simulink model "multi_rotor_sim"  (R2023b)
settings: Solver=ode4  StartTime=0.0  StopTime=inf  FixedStep=ST  RelTol=1e-3
values from neighbouring files (symbols this model uses):
  a0 = 0    [parameters.m]
  ASLOPE = 5.9    [parameters.m]
  Ax = 0.023    [parameters.m]
  Ay = 0.023    [parameters.m]
  Az = 0.106    [parameters.m]
  BLADES = 2    [parameters.m]
  BLCG = 0    [parameters.m]
  BLCP = 0    [parameters.m]
  BLH1 = b*sind(30)    [parameters.m]
  BLH2 = b    (= 0.275)    [parameters.m]
  BLH3 = b*sind(30)    [parameters.m]
  BLH4 = -b*sind(30)    [parameters.m]
  BLH5 = -b    (= -0.275)    [parameters.m]
  BLH6 = -b*sind(30)    [parameters.m]
  chi1 = 1    [parameters.m]
  chi2 = -1    [parameters.m]
  chi3 = 1    [parameters.m]
  chi4 = -1    [parameters.m]
  chi5 = 1    [parameters.m]
  chi6 = -1    [parameters.m]
  CHORD = 17.55e-3    (= 0.01755)    [parameters.m]
  CHORD75 = 21e-3    (= 0.021)    [parameters.m]
  dyn_viscosity = 17.89e-6    (= 1.789e-05)    [parameters.m]
  g0 = 9.80665    [parameters.m]
  href = 0    [parameters.m]
  k_ind = 1.35    [parameters.m]
  k_Omega = 14.92    [parameters.m]
  latref = 44.200626    [parameters.m]
  lonref = 12.063822    [parameters.m]
  m = 2.15    [parameters.m]
  MC_ATT_PITCH = 45*pi/180    (= 0.785398163397)    [parameters.m]
  MC_ATT_ROLL = 45*pi/180    (= 0.785398163397)    [parameters.m]
  MC_PITCH_P = 2    [parameters.m]
  MC_PITCHRATE_D = 0    [parameters.m]
  MC_PITCHRATE_I = 0.05    [parameters.m]
  MC_PITCHRATE_P = 0.09*3    (= 0.27)    [parameters.m]
  MC_RATE_PITCH = 500*pi/180    (= 8.72664625997)    [parameters.m]
  MC_RATE_ROLL = 500*pi/180    (= 8.72664625997)    [parameters.m]
  MC_RATE_YAW = 300*pi/180    (= 5.23598775598)    [parameters.m]
  MC_ROLL_P = 2    [parameters.m]
  MC_ROLLRATE_D = 0    [parameters.m]
  MC_ROLLRATE_I = 0.05    [parameters.m]
  MC_ROLLRATE_P = 0.09*3    (= 0.27)    [parameters.m]
  MC_VEL_FWD = 15    [parameters.m]
  MC_VEL_FWD_OPT = 0.5    [parameters.m]
  MC_VEL_LAT = 15    [parameters.m]
  MC_VEL_LAT_OPT = 0.5    [parameters.m]
  MC_VEL_VERT = 15    [parameters.m]
  MC_YAW_P = 0.55    [parameters.m]
  MC_YAWRATE_D = 0.05    [parameters.m]
  MC_YAWRATE_I = 0.02    [parameters.m]
  MC_YAWRATE_P = 0.15*3    (= 0.45)    [parameters.m]
  MPC_XY_VEL_D_ACC = 0.6    [parameters.m]
  MPC_XY_VEL_I_ACC = 0.8    [parameters.m]
  MPC_XY_VEL_P_ACC = 1.7    [parameters.m]
  MPC_Z_VEL_D_ACC = 0    [parameters.m]
  MPC_Z_VEL_I_ACC = 2    [parameters.m]
  MPC_Z_VEL_P_ACC = 4    [parameters.m]
  n = 0.6359    [parameters.m]
  p00 = 7.145e-2    (= 0.07145)    [parameters.m]
  p01 = 0.4377    [parameters.m]
  p02 = -10.13    [parameters.m]
  p10 = 1.259e-3    (= 0.001259)    [parameters.m]
  p11 = 1.284e-3    (= 0.001284)    [parameters.m]
  p20 = -7.513e-7    (= -7.513e-07)    [parameters.m]
  PWM_hover = (PWM_idle+PWM_max)/2    (= 1550)    [parameters.m]
  PWM_idle = 1100    [parameters.m]
  PWM_max = 2000    [parameters.m]
  ROTOR = 4*0.0254    (= 0.1016)    [parameters.m]
  ST = 0.01    [parameters.m]
  STACG = 0    [parameters.m]
  STACP = 0    [parameters.m]
  STAH1 = -b*cosd(30)    [parameters.m]
  STAH2 = 0    [parameters.m]
  STAH3 = b*cosd(30)    [parameters.m]
  STAH4 = b*cosd(30)    [parameters.m]
  STAH5 = 0    [parameters.m]
  STAH6 = -b*cosd(30)    [parameters.m]
  TERMINAL_SPEED = 0.5    [parameters.m]
  Theta0 = 45*pi/180    (= 0.785398163397)    [parameters.m]
  THETT = -38.0973*pi/180    (= -0.66492332112)    [parameters.m]
  wind_rate = [ 0 0 0 ]'    [parameters.m]
  wind_velocity_e = [ 0 0 0 ]'    [parameters.m]
  WLCG = -0.02    [parameters.m]
  WLCP = -0.08    [parameters.m]
  WLH1 = 32e-3    (= 0.032)    [parameters.m]
  WLH2 = 32e-3    (= 0.032)    [parameters.m]
  WLH3 = 32e-3    (= 0.032)    [parameters.m]
  WLH4 = 32e-3    (= 0.032)    [parameters.m]
  WLH5 = 32e-3    (= 0.032)    [parameters.m]
  WLH6 = 32e-3    (= 0.032)    [parameters.m]
undefined symbols (not defined in the file or in its folder): Earth, WGS84, X, Y, Z
libraries: sm_lib x258, slpidlib x36, nesl_utility x15, sharedtransform x13, aerolibutil x4, aerolibanimutils x3, sharedutil x2, sim3dlib x1, uavsim3dlib x1, shared6dof x1, aerolibtransform2 x1, aerolibatmos2 x1
(part 2 of 11)

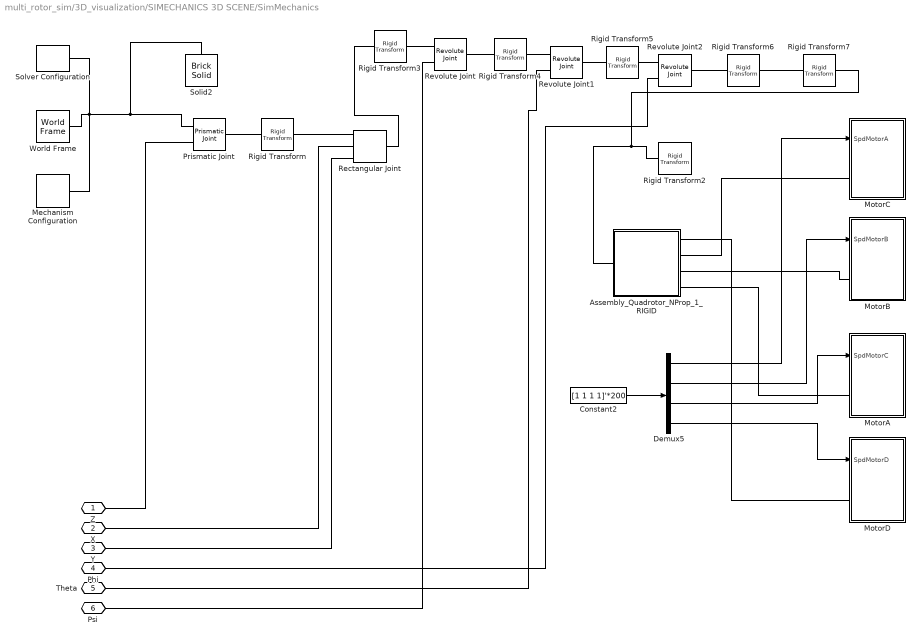
== system multi_rotor_sim/3D_visualization/SIMECHANICS 3D SCENE/SimMechanics ==
  Assembly_Quadrotor_NProp_1_RIGID : Subsystem
  Constant2 : Constant  Value=[1 1 1 1]'*200
  Demux5 : Demux
  Mechanism Configuration : sm_lib/Utilities/Mechanism Configuration  UniformGravity=Constant  GravityVector=[0 0 9.80665]  GravityVectorUnits=m/s^2  LinearizationDelta=0.001  JointModeTransitionNonlinearIterations=2
  MotorA : Subsystem
  MotorB : Subsystem
  MotorC : Subsystem
  MotorD : Subsystem
  Prismatic Joint : sm_lib/Joints/Prismatic Joint  JointMode=Normal  SenseConstraintForce=off  SenseConstraintForceX=off  SenseConstraintForceY=off  SenseConstraintForceZ=off  SenseConstraintTorque=off  SenseConstraintTorqueX=off  SenseConstraintTorqueY=off  SenseConstraintTorqueZ=off  SenseTotalForce=off  SenseTotalForceX=off  SenseTotalForceY=off  SenseTotalForceZ=off  SenseTotalTorque=off  SenseTotalTorqueX=off  SenseTotalTorqueY=off  SenseTotalTorqueZ=off  CompositeWrenchDir=FollowerOnBase  CompositeWrenchFrame=BaseFrame  EquilibriumPosition=0  EquilibriumPositionUnits=m  SpringStiffness=0  SpringStiffnessUnits=N/m  DampingCoefficient=0  DampingCoefficientUnits=N/(m/s)  TorqueActuationMode=ComputedTorque  MotionActuationMode=InputMotion  SensePosition=off  SenseVelocity=off  SenseAcceleration=off  SenseTorqueForce=off  SenseLowerLimitTorqueForce=off  SenseUpperLimitTorqueForce=off  LowerLimitSpecify=off  LowerLimitBound=-1  LowerLimitBoundUnits=m  LowerLimitStiffness=1e6  LowerLimitStiffnessUnits=N/m  LowerLimitDamping=1e3  LowerLimitDampingUnits=N/(m/s)  LowerLimitTransitionRegionWidth=1e-4  LowerLimitTransitionRegionWidthUnits=m  UpperLimitSpecify=off  UpperLimitBound=1  UpperLimitBoundUnits=m  UpperLimitStiffness=1e6  UpperLimitStiffnessUnits=N/m  UpperLimitDamping=1e3  UpperLimitDampingUnits=N/(m/s)  UpperLimitTransitionRegionWidth=1e-4  UpperLimitTransitionRegionWidthUnits=m  PositionTargetSpecify=off  PositionTargetPriority=High  PositionTargetValue=0  PositionTargetValueUnits=m  VelocityTargetSpecify=off  VelocityTargetPriority=High  VelocityTargetValue=0  VelocityTargetValueUnits=m/s
  Rectangular Joint : sm_lib/Joints/Rectangular Joint  JointMode=Normal  SenseConstraintForce=off  SenseConstraintForceX=off  SenseConstraintForceY=off  SenseConstraintForceZ=off  SenseConstraintTorque=off  SenseConstraintTorqueX=off  SenseConstraintTorqueY=off  SenseConstraintTorqueZ=off  SenseTotalForce=off  SenseTotalForceX=off  SenseTotalForceY=off  SenseTotalForceZ=off  SenseTotalTorque=off  SenseTotalTorqueX=off  SenseTotalTorqueY=off  SenseTotalTorqueZ=off  CompositeWrenchDir=FollowerOnBase  CompositeWrenchFrame=BaseFrame  PxEquilibriumPosition=0  PxEquilibriumPositionUnits=m  PxSpringStiffness=0  PxSpringStiffnessUnits=N/m  PxDampingCoefficient=0  PxDampingCoefficientUnits=N/(m/s)  PxTorqueActuationMode=ComputedTorque  PxMotionActuationMode=InputMotion  PxSensePosition=off  PxSenseVelocity=off  PxSenseAcceleration=off  PxSenseTorqueForce=off  PxSenseLowerLimitTorqueForce=off  PxSenseUpperLimitTorqueForce=off  PxLowerLimitSpecify=off  PxLowerLimitBound=-1  PxLowerLimitBoundUnits=m  PxLowerLimitStiffness=1e6  PxLowerLimitStiffnessUnits=N/m  PxLowerLimitDamping=1e3  PxLowerLimitDampingUnits=N/(m/s)  PxLowerLimitTransitionRegionWidth=1e-4  PxLowerLimitTransitionRegionWidthUnits=m  PxUpperLimitSpecify=off  PxUpperLimitBound=1  PxUpperLimitBoundUnits=m  PxUpperLimitStiffness=1e6  PxUpperLimitStiffnessUnits=N/m  PxUpperLimitDamping=1e3  PxUpperLimitDampingUnits=N/(m/s)  PxUpperLimitTransitionRegionWidth=1e-4  PxUpperLimitTransitionRegionWidthUnits=m  PxPositionTargetSpecify=off  PxPositionTargetPriority=High  PxPositionTargetValue=0  PxPositionTargetValueUnits=m  PxVelocityTargetSpecify=off  PxVelocityTargetPriority=High  PxVelocityTargetValue=0  PxVelocityTargetValueUnits=m/s  PyEquilibriumPosition=0  PyEquilibriumPositionUnits=m  PySpringStiffness=0  PySpringStiffnessUnits=N/m  PyDampingCoefficient=0  PyDampingCoefficientUnits=N/(m/s)  PyTorqueActuationMode=ComputedTorque  PyMotionActuationMode=InputMotion  PySensePosition=off  PySenseVelocity=off  PySenseAcceleration=off  PySenseTorqueForce=off  PySenseLowerLimitTorqueForce=off  PySenseUpperLimitTorqueForce=off  PyLowerLimitSpecify=off  PyLowerLimitBound=-1  PyLowerLimitBoundUnits=m  PyLowerLimitStiffness=1e6  PyLowerLimitStiffnessUnits=N/m  PyLowerLimitDamping=1e3  PyLowerLimitDampingUnits=N/(m/s)  PyLowerLimitTransitionRegionWidth=1e-4  PyLowerLimitTransitionRegionWidthUnits=m  PyUpperLimitSpecify=off  PyUpperLimitBound=1  PyUpperLimitBoundUnits=m  PyUpperLimitStiffness=1e6  PyUpperLimitStiffnessUnits=N/m  PyUpperLimitDamping=1e3  PyUpperLimitDampingUnits=N/(m/s)  PyUpperLimitTransitionRegionWidth=1e-4  PyUpperLimitTransitionRegionWidthUnits=m  PyPositionTargetSpecify=off  PyPositionTargetPriority=High  PyPositionTargetValue=0  PyPositionTargetValueUnits=m  PyVelocityTargetSpecify=off  PyVelocityTargetPriority=High  PyVelocityTargetValue=0  PyVelocityTargetValueUnits=m/s
  Revolute Joint : sm_lib/Joints/Revolute Joint  JointMode=Normal  SenseConstraintForce=off  SenseConstraintForceX=off  SenseConstraintForceY=off  SenseConstraintForceZ=off  SenseConstraintTorque=off  SenseConstraintTorqueX=off  SenseConstraintTorqueY=off  SenseConstraintTorqueZ=off  SenseTotalForce=off  SenseTotalForceX=off  SenseTotalForceY=off  SenseTotalForceZ=off  SenseTotalTorque=off  SenseTotalTorqueX=off  SenseTotalTorqueY=off  SenseTotalTorqueZ=off  CompositeWrenchDir=FollowerOnBase  CompositeWrenchFrame=BaseFrame  EquilibriumPosition=0  EquilibriumPositionUnits=deg  SpringStiffness=0  SpringStiffnessUnits=N*m/deg  DampingCoefficient=0  DampingCoefficientUnits=N*m/(deg/s)  TorqueActuationMode=ComputedTorque  MotionActuationMode=InputMotion  SensePosition=off  SenseVelocity=off  SenseAcceleration=off  SenseTorqueForce=off  SenseLowerLimitTorqueForce=off  SenseUpperLimitTorqueForce=off  LowerLimitSpecify=off  LowerLimitBound=-90  LowerLimitBoundUnits=deg  LowerLimitStiffness=1e4  LowerLimitStiffnessUnits=N*m/deg  LowerLimitDamping=10  LowerLimitDampingUnits=N*m/(deg/s)  LowerLimitTransitionRegionWidth=0.1  LowerLimitTransitionRegionWidthUnits=deg  UpperLimitSpecify=off  UpperLimitBound=90  UpperLimitBoundUnits=deg  UpperLimitStiffness=1e4  UpperLimitStiffnessUnits=N*m/deg  UpperLimitDamping=10  UpperLimitDampingUnits=N*m/(deg/s)  UpperLimitTransitionRegionWidth=0.1  UpperLimitTransitionRegionWidthUnits=deg  PositionTargetSpecify=off  PositionTargetPriority=High  PositionTargetValue=0  PositionTargetValueUnits=deg  VelocityTargetSpecify=off  VelocityTargetPriority=High  VelocityTargetValue=0  VelocityTargetValueUnits=deg/s
  Revolute Joint1 : sm_lib/Joints/Revolute Joint  JointMode=Normal  SenseConstraintForce=off  SenseConstraintForceX=off  SenseConstraintForceY=off  SenseConstraintForceZ=off  SenseConstraintTorque=off  SenseConstraintTorqueX=off  SenseConstraintTorqueY=off  SenseConstraintTorqueZ=off  SenseTotalForce=off  SenseTotalForceX=off  SenseTotalForceY=off  SenseTotalForceZ=off  SenseTotalTorque=off  SenseTotalTorqueX=off  SenseTotalTorqueY=off  SenseTotalTorqueZ=off  CompositeWrenchDir=FollowerOnBase  CompositeWrenchFrame=BaseFrame  EquilibriumPosition=0  EquilibriumPositionUnits=deg  SpringStiffness=0  SpringStiffnessUnits=N*m/deg  DampingCoefficient=0  DampingCoefficientUnits=N*m/(deg/s)  TorqueActuationMode=ComputedTorque  MotionActuationMode=InputMotion  SensePosition=off  SenseVelocity=off  SenseAcceleration=off  SenseTorqueForce=off  SenseLowerLimitTorqueForce=off  SenseUpperLimitTorqueForce=off  LowerLimitSpecify=off  LowerLimitBound=-90  LowerLimitBoundUnits=deg  LowerLimitStiffness=1e4  LowerLimitStiffnessUnits=N*m/deg  LowerLimitDamping=10  LowerLimitDampingUnits=N*m/(deg/s)  LowerLimitTransitionRegionWidth=0.1  LowerLimitTransitionRegionWidthUnits=deg  UpperLimitSpecify=off  UpperLimitBound=90  UpperLimitBoundUnits=deg  UpperLimitStiffness=1e4  UpperLimitStiffnessUnits=N*m/deg  UpperLimitDamping=10  UpperLimitDampingUnits=N*m/(deg/s)  UpperLimitTransitionRegionWidth=0.1  UpperLimitTransitionRegionWidthUnits=deg  PositionTargetSpecify=off  PositionTargetPriority=High  PositionTargetValue=0  PositionTargetValueUnits=deg  VelocityTargetSpecify=off  VelocityTargetPriority=High  VelocityTargetValue=0  VelocityTargetValueUnits=deg/s
  Revolute Joint2 : sm_lib/Joints/Revolute Joint  JointMode=Normal  SenseConstraintForce=off  SenseConstraintForceX=off  SenseConstraintForceY=off  SenseConstraintForceZ=off  SenseConstraintTorque=off  SenseConstraintTorqueX=off  SenseConstraintTorqueY=off  SenseConstraintTorqueZ=off  SenseTotalForce=off  SenseTotalForceX=off  SenseTotalForceY=off  SenseTotalForceZ=off  SenseTotalTorque=off  SenseTotalTorqueX=off  SenseTotalTorqueY=off  SenseTotalTorqueZ=off  CompositeWrenchDir=FollowerOnBase  CompositeWrenchFrame=BaseFrame  EquilibriumPosition=0  EquilibriumPositionUnits=deg  SpringStiffness=0  SpringStiffnessUnits=N*m/deg  DampingCoefficient=0  DampingCoefficientUnits=N*m/(deg/s)  TorqueActuationMode=ComputedTorque  MotionActuationMode=InputMotion  SensePosition=off  SenseVelocity=off  SenseAcceleration=off  SenseTorqueForce=off  SenseLowerLimitTorqueForce=off  SenseUpperLimitTorqueForce=off  LowerLimitSpecify=off  LowerLimitBound=-90  LowerLimitBoundUnits=deg  LowerLimitStiffness=1e4  LowerLimitStiffnessUnits=N*m/deg  LowerLimitDamping=10  LowerLimitDampingUnits=N*m/(deg/s)  LowerLimitTransitionRegionWidth=0.1  LowerLimitTransitionRegionWidthUnits=deg  UpperLimitSpecify=off  UpperLimitBound=90  UpperLimitBoundUnits=deg  UpperLimitStiffness=1e4  UpperLimitStiffnessUnits=N*m/deg  UpperLimitDamping=10  UpperLimitDampingUnits=N*m/(deg/s)  UpperLimitTransitionRegionWidth=0.1  UpperLimitTransitionRegionWidthUnits=deg  PositionTargetSpecify=off  PositionTargetPriority=High  PositionTargetValue=0  PositionTargetValueUnits=deg  VelocityTargetSpecify=off  VelocityTargetPriority=High  VelocityTargetValue=0  VelocityTargetValueUnits=deg/s
  Rigid Transform : sm_lib/Frames and Transforms/Rigid Transform  TranslationMethod=None  TranslationStandardOffset=0  TranslationStandardOffsetUnits=m  TranslationStandardAxis=+Z  TranslationCartesianOffset=[0 0 0]  TranslationCartesianOffsetUnits=m  TranslationROffset=0  TranslationROffsetUnits=m  TranslationZOffset=0  TranslationZOffsetUnits=m  TranslationThetaOffset=0  TranslationThetaOffsetUnits=deg  RotationMethod=None  RotationAngleUnits=deg  RotationStandardAxis=+Z  RotationAngle=0.0  RotationArbitraryAxis=[0 0 1]  FollAlignAxisA=+X  BaseAlignAxisA=+Y  FollAlignAxisB=+Y  BaseAlignAxisB=+Z  RotationSequenceAxes=FollowerAxes  RotationSequence=XYX  RotationSequenceAngles=[0 0 0]  RotationSequenceAnglesUnits=deg  RotationMatrix=[1 0 0; 0 1 0; 0 0 1]  Quaternion=[1 0 0 0]
  Rigid Transform2 : sm_lib/Frames and Transforms/Rigid Transform  TranslationMethod=None  TranslationStandardOffset=0  TranslationStandardOffsetUnits=m  TranslationStandardAxis=+Z  TranslationCartesianOffset=[0 0 0]  TranslationCartesianOffsetUnits=m  TranslationROffset=0  TranslationROffsetUnits=m  TranslationZOffset=0  TranslationZOffsetUnits=m  TranslationThetaOffset=0  TranslationThetaOffsetUnits=deg  RotationMethod=None  RotationAngleUnits=deg  RotationStandardAxis=+Z  RotationAngle=0.0  RotationArbitraryAxis=[0 0 1]  FollAlignAxisA=+X  BaseAlignAxisA=+Y  FollAlignAxisB=+Y  BaseAlignAxisB=+Z  RotationSequenceAxes=FollowerAxes  RotationSequence=XYX  RotationSequenceAngles=[0 0 0]  RotationSequenceAnglesUnits=deg  RotationMatrix=[1 0 0; 0 1 0; 0 0 1]  Quaternion=[1 0 0 0]
  Rigid Transform3 : sm_lib/Frames and Transforms/Rigid Transform  TranslationMethod=None  TranslationStandardOffset=0  TranslationStandardOffsetUnits=m  TranslationStandardAxis=+Z  TranslationCartesianOffset=[0 0 0]  TranslationCartesianOffsetUnits=m  TranslationROffset=0  TranslationROffsetUnits=m  TranslationZOffset=0  TranslationZOffsetUnits=m  TranslationThetaOffset=0  TranslationThetaOffsetUnits=deg  RotationMethod=None  RotationAngleUnits=deg  RotationStandardAxis=+Z  RotationAngle=0.0  RotationArbitraryAxis=[0 0 1]  FollAlignAxisA=+X  BaseAlignAxisA=+Y  FollAlignAxisB=+Y  BaseAlignAxisB=+Z  RotationSequenceAxes=FollowerAxes  RotationSequence=XYX  RotationSequenceAngles=[0 0 0]  RotationSequenceAnglesUnits=deg  RotationMatrix=[1 0 0; 0 1 0; 0 0 1]  Quaternion=[1 0 0 0]
  Rigid Transform4 : sm_lib/Frames and Transforms/Rigid Transform  TranslationMethod=None  TranslationStandardOffset=0  TranslationStandardOffsetUnits=m  TranslationStandardAxis=+Z  TranslationCartesianOffset=[0 0 0]  TranslationCartesianOffsetUnits=m  TranslationROffset=0  TranslationROffsetUnits=m  TranslationZOffset=0  TranslationZOffsetUnits=m  TranslationThetaOffset=0  TranslationThetaOffsetUnits=deg  RotationMethod=ArbitraryAxis  RotationAngleUnits=deg  RotationStandardAxis=+Z  RotationAngle=-90  RotationArbitraryAxis=[1 0 0]  FollAlignAxisA=+X  BaseAlignAxisA=+Y  FollAlignAxisB=+Y  BaseAlignAxisB=+Z  RotationSequenceAxes=FollowerAxes  RotationSequence=XYX  RotationSequenceAngles=[0 0 0]  RotationSequenceAnglesUnits=deg  RotationMatrix=[1 0 0; 0 1 0; 0 0 1]  Quaternion=[1 0 0 0]
  Rigid Transform5 : sm_lib/Frames and Transforms/Rigid Transform  TranslationMethod=None  TranslationStandardOffset=0  TranslationStandardOffsetUnits=m  TranslationStandardAxis=+Z  TranslationCartesianOffset=[0 0 0]  TranslationCartesianOffsetUnits=m  TranslationROffset=0  TranslationROffsetUnits=m  TranslationZOffset=0  TranslationZOffsetUnits=m  TranslationThetaOffset=0  TranslationThetaOffsetUnits=deg  RotationMethod=ArbitraryAxis  RotationAngleUnits=deg  RotationStandardAxis=+Z  RotationAngle=90  RotationArbitraryAxis=[0 1 0]  FollAlignAxisA=+X  BaseAlignAxisA=+Y  FollAlignAxisB=+Y  BaseAlignAxisB=+Z  RotationSequenceAxes=FollowerAxes  RotationSequence=XYX  RotationSequenceAngles=[0 0 0]  RotationSequenceAnglesUnits=deg  RotationMatrix=[1 0 0; 0 1 0; 0 0 1]  Quaternion=[1 0 0 0]
  Rigid Transform6 : sm_lib/Frames and Transforms/Rigid Transform  TranslationMethod=None  TranslationStandardOffset=0  TranslationStandardOffsetUnits=m  TranslationStandardAxis=+Z  TranslationCartesianOffset=[0 0 0]  TranslationCartesianOffsetUnits=m  TranslationROffset=0  TranslationROffsetUnits=m  TranslationZOffset=0  TranslationZOffsetUnits=m  TranslationThetaOffset=0  TranslationThetaOffsetUnits=deg  RotationMethod=ArbitraryAxis  RotationAngleUnits=deg  RotationStandardAxis=+Z  RotationAngle=-90  RotationArbitraryAxis=[0 1 0]  FollAlignAxisA=+X  BaseAlignAxisA=+Y  FollAlignAxisB=+Y  BaseAlignAxisB=+Z  RotationSequenceAxes=FollowerAxes  RotationSequence=XYX  RotationSequenceAngles=[0 0 0]  RotationSequenceAnglesUnits=deg  RotationMatrix=[1 0 0; 0 1 0; 0 0 1]  Quaternion=[1 0 0 0]
  Rigid Transform7 : sm_lib/Frames and Transforms/Rigid Transform  TranslationMethod=None  TranslationStandardOffset=0  TranslationStandardOffsetUnits=m  TranslationStandardAxis=+Z  TranslationCartesianOffset=[0 0 0]  TranslationCartesianOffsetUnits=m  TranslationROffset=0  TranslationROffsetUnits=m  TranslationZOffset=0  TranslationZOffsetUnits=m  TranslationThetaOffset=0  TranslationThetaOffsetUnits=deg  RotationMethod=ArbitraryAxis  RotationAngleUnits=deg  RotationStandardAxis=+Z  RotationAngle=90  RotationArbitraryAxis=[1 0 0]  FollAlignAxisA=+X  BaseAlignAxisA=+Y  FollAlignAxisB=+Y  BaseAlignAxisB=+Z  RotationSequenceAxes=FollowerAxes  RotationSequence=XYX  RotationSequenceAngles=[0 0 0]  RotationSequenceAnglesUnits=deg  RotationMatrix=[1 0 0; 0 1 0; 0 0 1]  Quaternion=[1 0 0 0]
  Solid2 : sm_lib/Body Elements/Brick Solid  GraphicAmbientColor=[0.15 0.15 0.15 1.0]  BasedOnType=Density  BrickDimensions=[10 10 0.01]  BrickDimensionsUnits=m  CenterOfMass=[0 0 0]  CenterOfMassUnits=m  GraphicDiffuseColor=[0.6 1.0 0.6]  Density=1000  DensityUnits=kg/(m^3)  DoExposeReferenceFrame=on  GraphicEmissiveColor=[0.0 0.0 0.0 1.0]  ExportEntireGeometry=off  SerializedFrames=<Frames/>  MarkerShape=Sphere  MarkerSize=10  GraphicType=FromGeometry  InertiaType=CalculateFromGeometry  Mass=1  MassUnits=kg  MomentsOfInertia=[1 1 1]  MomentsOfInertiaUnits=kg*m^2  GraphicOpacity=1.0  ProductsOfInertia=[0 0 0]  ProductsOfInertiaUnits=kg*m^2  GraphicShininess=75  GraphicSpecularColor=[0.5 0.5 0.5 1.0]  GraphicVisPropType=SimpleVisualProperties
  Solver Configuration : nesl_utility/Solver Configuration  PhysicalDomain=network_engine_domain  SubClassName=solver  LeftPortType=input  RightPortType=generic  Tones=[]  Harmonics=[]  SimulateNoise=off  Profile=off  UseLocalSampling=off  EnableSwitchedLinearOptims=on  FrequencyDomain=off  UseCCode=off  RelTol=0.001  AbsTol=1e-06  MinStep=1e-09  ToWorkspace=off  RevertToSquareIcSolve=off  NumHomotopyIterations=100  PhasorMode=off  PhasorModeNumHarmonics=1  ConsistencySolver=NEWTON_FTOL  IndexReductionMethod=DerivativeReplacement  DoDC=off  ResidualTolerance=1e-09  ConsistencyTolSource=GLOBAL  ConsistencyAbsTol=0.001  ConsistencyRelTol=0.001  ConsistencyTolFactor=0.001  UseLocalSolver=off  LocalSolverChoice=NE_BACKWARD_EULER_ADVANCER  ResolveIndetEquations=on  FunctionEvalNumThread=1  LocalSolverSampleTime=0.001  DoFixedCost=off  MaxNonlinIter=3  MaxModeIter=2  ComputeImpulses=off  ImpulseIterations=2  LinearAlgebra=Sparse  LinearAlgebraNumThread=0  EquationFormulation=NE_TIME_EF  DelaysMemoryBudget=1024  AutomaticFiltering=on  FilteringTimeConstant=0.001  PartitionStorageMethod=AS_NEEDED  PartitionMemoryBudget=1024  PartitionMethod=FAST  MultibodyUseLocalSolver=off  MultibodyLocalSolverChoice=ODE1  MultibodyLocalSolverSampleTime=0.001
  World Frame : sm_lib/Frames and Transforms/World Frame
  Z : PMIOPort  Side=Left
  X : PMIOPort  Port=2  Side=Left
  Y : PMIOPort  Port=3  Side=Left
  Phi : PMIOPort  Port=4  Side=Left
  Theta : PMIOPort  Port=5  Side=Left
  Psi : PMIOPort  Port=6  Side=Left
  wires:
  Constant2/1 -> Demux5/1
  Demux5/4 -> MotorD/1(SpdMotorD)
  Demux5/3 -> MotorA/1(SpdMotorC)
  Demux5/2 -> MotorB/1(SpdMotorB)
  Demux5/1 -> MotorC/1(SpdMotorA)
  connections:
  Rigid Transform6/RConn1 -- Rigid Transform7/LConn1
  Revolute Joint2/RConn1 -- Rigid Transform6/LConn1
  Revolute Joint1/RConn1 -- Rigid Transform5/LConn1
  Revolute Joint/RConn1 -- Rigid Transform4/LConn1
  Rigid Transform3/RConn1 -- Revolute Joint/LConn1
  Rigid Transform4/RConn1 -- Revolute Joint1/LConn1
  Revolute Joint2/LConn1 -- Rigid Transform5/RConn1
  Assembly_Quadrotor_NProp_1_RIGID/RConn1 -- MotorD/LConn1
  Assembly_Quadrotor_NProp_1_RIGID/RConn2 -- MotorC/LConn1
  Assembly_Quadrotor_NProp_1_RIGID/RConn3 -- MotorB/LConn1
  Assembly_Quadrotor_NProp_1_RIGID/RConn4 -- MotorA/LConn1
  Psi/RConn1 -- Revolute Joint/LConn2
  Theta/RConn1 -- Revolute Joint1/LConn2
  Y/RConn1 -- Rectangular Joint/LConn3
  Phi/RConn1 -- Revolute Joint2/LConn2
  X/RConn1 -- Rectangular Joint/LConn2
  Z/RConn1 -- Prismatic Joint/LConn2
  Rigid Transform2/LConn1 -- Rigid Transform7/RConn1 -- Assembly_Quadrotor_NProp_1_RIGID/LConn1
  Rectangular Joint/RConn1 -- Rigid Transform3/LConn1
  Rigid Transform/RConn1 -- Rectangular Joint/LConn1
  Rigid Transform/LConn1 -- Prismatic Joint/RConn1
  Prismatic Joint/LConn1 -- Solid2/RConn1 -- Solver Configuration/RConn1 -- Mechanism Configuration/RConn1 -- World Frame/RConn1

== system multi_rotor_sim/3D_visualization/SIMECHANICS 3D SCENE/SimMechanics1 ==
  Mechanism Configuration : sm_lib/Utilities/Mechanism Configuration  UniformGravity=Constant  GravityVector=[0 0 9.80665]  GravityVectorUnits=m/s^2  LinearizationDelta=0.001  JointModeTransitionNonlinearIterations=2
  Prismatic Joint : sm_lib/Joints/Prismatic Joint  JointMode=Normal  SenseConstraintForce=off  SenseConstraintForceX=off  SenseConstraintForceY=off  SenseConstraintForceZ=off  SenseConstraintTorque=off  SenseConstraintTorqueX=off  SenseConstraintTorqueY=off  SenseConstraintTorqueZ=off  SenseTotalForce=off  SenseTotalForceX=off  SenseTotalForceY=off  SenseTotalForceZ=off  SenseTotalTorque=off  SenseTotalTorqueX=off  SenseTotalTorqueY=off  SenseTotalTorqueZ=off  CompositeWrenchDir=FollowerOnBase  CompositeWrenchFrame=BaseFrame  EquilibriumPosition=0  EquilibriumPositionUnits=m  SpringStiffness=0  SpringStiffnessUnits=N/m  DampingCoefficient=0  DampingCoefficientUnits=N/(m/s)  TorqueActuationMode=ComputedTorque  MotionActuationMode=InputMotion  SensePosition=off  SenseVelocity=off  SenseAcceleration=off  SenseTorqueForce=off  SenseLowerLimitTorqueForce=off  SenseUpperLimitTorqueForce=off  LowerLimitSpecify=off  LowerLimitBound=-1  LowerLimitBoundUnits=m  LowerLimitStiffness=1e6  LowerLimitStiffnessUnits=N/m  LowerLimitDamping=1e3  LowerLimitDampingUnits=N/(m/s)  LowerLimitTransitionRegionWidth=1e-4  LowerLimitTransitionRegionWidthUnits=m  UpperLimitSpecify=off  UpperLimitBound=1  UpperLimitBoundUnits=m  UpperLimitStiffness=1e6  UpperLimitStiffnessUnits=N/m  UpperLimitDamping=1e3  UpperLimitDampingUnits=N/(m/s)  UpperLimitTransitionRegionWidth=1e-4  UpperLimitTransitionRegionWidthUnits=m  PositionTargetSpecify=off  PositionTargetPriority=High  PositionTargetValue=0  PositionTargetValueUnits=m  VelocityTargetSpecify=off  VelocityTargetPriority=High  VelocityTargetValue=0  VelocityTargetValueUnits=m/s
  Rectangular Joint : sm_lib/Joints/Rectangular Joint  JointMode=Normal  SenseConstraintForce=off  SenseConstraintForceX=off  SenseConstraintForceY=off  SenseConstraintForceZ=off  SenseConstraintTorque=off  SenseConstraintTorqueX=off  SenseConstraintTorqueY=off  SenseConstraintTorqueZ=off  SenseTotalForce=off  SenseTotalForceX=off  SenseTotalForceY=off  SenseTotalForceZ=off  SenseTotalTorque=off  SenseTotalTorqueX=off  SenseTotalTorqueY=off  SenseTotalTorqueZ=off  CompositeWrenchDir=FollowerOnBase  CompositeWrenchFrame=BaseFrame  PxEquilibriumPosition=0  PxEquilibriumPositionUnits=m  PxSpringStiffness=0  PxSpringStiffnessUnits=N/m  PxDampingCoefficient=0  PxDampingCoefficientUnits=N/(m/s)  PxTorqueActuationMode=ComputedTorque  PxMotionActuationMode=InputMotion  PxSensePosition=off  PxSenseVelocity=off  PxSenseAcceleration=off  PxSenseTorqueForce=off  PxSenseLowerLimitTorqueForce=off  PxSenseUpperLimitTorqueForce=off  PxLowerLimitSpecify=off  PxLowerLimitBound=-1  PxLowerLimitBoundUnits=m  PxLowerLimitStiffness=1e6  PxLowerLimitStiffnessUnits=N/m  PxLowerLimitDamping=1e3  PxLowerLimitDampingUnits=N/(m/s)  PxLowerLimitTransitionRegionWidth=1e-4  PxLowerLimitTransitionRegionWidthUnits=m  PxUpperLimitSpecify=off  PxUpperLimitBound=1  PxUpperLimitBoundUnits=m  PxUpperLimitStiffness=1e6  PxUpperLimitStiffnessUnits=N/m  PxUpperLimitDamping=1e3  PxUpperLimitDampingUnits=N/(m/s)  PxUpperLimitTransitionRegionWidth=1e-4  PxUpperLimitTransitionRegionWidthUnits=m  PxPositionTargetSpecify=off  PxPositionTargetPriority=High  PxPositionTargetValue=0  PxPositionTargetValueUnits=m  PxVelocityTargetSpecify=off  PxVelocityTargetPriority=High  PxVelocityTargetValue=0  PxVelocityTargetValueUnits=m/s  PyEquilibriumPosition=0  PyEquilibriumPositionUnits=m  PySpringStiffness=0  PySpringStiffnessUnits=N/m  PyDampingCoefficient=0  PyDampingCoefficientUnits=N/(m/s)  PyTorqueActuationMode=ComputedTorque  PyMotionActuationMode=InputMotion  PySensePosition=off  PySenseVelocity=off  PySenseAcceleration=off  PySenseTorqueForce=off  PySenseLowerLimitTorqueForce=off  PySenseUpperLimitTorqueForce=off  PyLowerLimitSpecify=off  PyLowerLimitBound=-1  PyLowerLimitBoundUnits=m  PyLowerLimitStiffness=1e6  PyLowerLimitStiffnessUnits=N/m  PyLowerLimitDamping=1e3  PyLowerLimitDampingUnits=N/(m/s)  PyLowerLimitTransitionRegionWidth=1e-4  PyLowerLimitTransitionRegionWidthUnits=m  PyUpperLimitSpecify=off  PyUpperLimitBound=1  PyUpperLimitBoundUnits=m  PyUpperLimitStiffness=1e6  PyUpperLimitStiffnessUnits=N/m  PyUpperLimitDamping=1e3  PyUpperLimitDampingUnits=N/(m/s)  PyUpperLimitTransitionRegionWidth=1e-4  PyUpperLimitTransitionRegionWidthUnits=m  PyPositionTargetSpecify=off  PyPositionTargetPriority=High  PyPositionTargetValue=0  PyPositionTargetValueUnits=m  PyVelocityTargetSpecify=off  PyVelocityTargetPriority=High  PyVelocityTargetValue=0  PyVelocityTargetValueUnits=m/s
  Rigid Transform : sm_lib/Frames and Transforms/Rigid Transform  TranslationMethod=None  TranslationStandardOffset=0  TranslationStandardOffsetUnits=m  TranslationStandardAxis=+Z  TranslationCartesianOffset=[0 0 0]  TranslationCartesianOffsetUnits=m  TranslationROffset=0  TranslationROffsetUnits=m  TranslationZOffset=0  TranslationZOffsetUnits=m  TranslationThetaOffset=0  TranslationThetaOffsetUnits=deg  RotationMethod=None  RotationAngleUnits=deg  RotationStandardAxis=+Z  RotationAngle=0.0  RotationArbitraryAxis=[0 0 1]  FollAlignAxisA=+X  BaseAlignAxisA=+Y  FollAlignAxisB=+Y  BaseAlignAxisB=+Z  RotationSequenceAxes=FollowerAxes  RotationSequence=XYX  RotationSequenceAngles=[0 0 0]  RotationSequenceAnglesUnits=deg  RotationMatrix=[1 0 0; 0 1 0; 0 0 1]  Quaternion=[1 0 0 0]
  Solid1 : sm_lib/Body Elements/Spherical Solid  GraphicAmbientColor=[0.15 0.15 0.15 1.0]  BasedOnType=Density  CenterOfMass=[0 0 0]  CenterOfMassUnits=m  GraphicDiffuseColor=[1.0 0.0 0.0]  Density=1000  DensityUnits=kg/(m^3)  DoExposeReferenceFrame=on  GraphicEmissiveColor=[0.0 0.0 0.0 1.0]  ExportEntireGeometry=off  SerializedExposedGeometries=<ExposedGeometries/>  SerializedFrames=<Frames/>  MarkerShape=Sphere  MarkerSize=10  GraphicType=FromGeometry  InertiaType=CalculateFromGeometry  Mass=1  MassUnits=kg  MomentsOfInertia=[1 1 1]  MomentsOfInertiaUnits=kg*m^2  GraphicOpacity=0.5  ProductsOfInertia=[0 0 0]  ProductsOfInertiaUnits=kg*m^2  GraphicShininess=75  GraphicSpecularColor=[0.5 0.5 0.5 1.0]  SphereRadius=0.05  SphereRadiusUnits=m  GraphicVisPropType=SimpleVisualProperties
  Solver Configuration : nesl_utility/Solver Configuration  PhysicalDomain=network_engine_domain  SubClassName=solver  LeftPortType=input  RightPortType=generic  Tones=[]  Harmonics=[]  SimulateNoise=off  Profile=off  UseLocalSampling=off  EnableSwitchedLinearOptims=on  FrequencyDomain=off  UseCCode=off  RelTol=0.001  AbsTol=1e-06  MinStep=1e-09  ToWorkspace=off  RevertToSquareIcSolve=off  NumHomotopyIterations=100  PhasorMode=off  PhasorModeNumHarmonics=1  ConsistencySolver=NEWTON_FTOL  IndexReductionMethod=DerivativeReplacement  DoDC=off  ResidualTolerance=1e-09  ConsistencyTolSource=GLOBAL  ConsistencyAbsTol=0.001  ConsistencyRelTol=0.001  ConsistencyTolFactor=0.001  UseLocalSolver=off  LocalSolverChoice=NE_BACKWARD_EULER_ADVANCER  ResolveIndetEquations=on  FunctionEvalNumThread=1  LocalSolverSampleTime=0.001  DoFixedCost=off  MaxNonlinIter=3  MaxModeIter=2  ComputeImpulses=off  ImpulseIterations=2  LinearAlgebra=Sparse  LinearAlgebraNumThread=0  EquationFormulation=NE_TIME_EF  DelaysMemoryBudget=1024  AutomaticFiltering=on  FilteringTimeConstant=0.001  PartitionStorageMethod=AS_NEEDED  PartitionMemoryBudget=1024  PartitionMethod=FAST  MultibodyUseLocalSolver=off  MultibodyLocalSolverChoice=ODE1  MultibodyLocalSolverSampleTime=0.001
  World Frame : sm_lib/Frames and Transforms/World Frame
  Z : PMIOPort  Side=Left
  X : PMIOPort  Port=2  Side=Left
  Y : PMIOPort  Port=3  Side=Left
  connections:
  World Frame/RConn1 -- Prismatic Joint/LConn1 -- Mechanism Configuration/RConn1 -- Solver Configuration/RConn1
  Rigid Transform/LConn1 -- Prismatic Joint/RConn1
  Rigid Transform/RConn1 -- Rectangular Joint/LConn1
  Rectangular Joint/RConn1 -- Solid1/RConn1
  Z/RConn1 -- Prismatic Joint/LConn2
  X/RConn1 -- Rectangular Joint/LConn2
  Y/RConn1 -- Rectangular Joint/LConn3

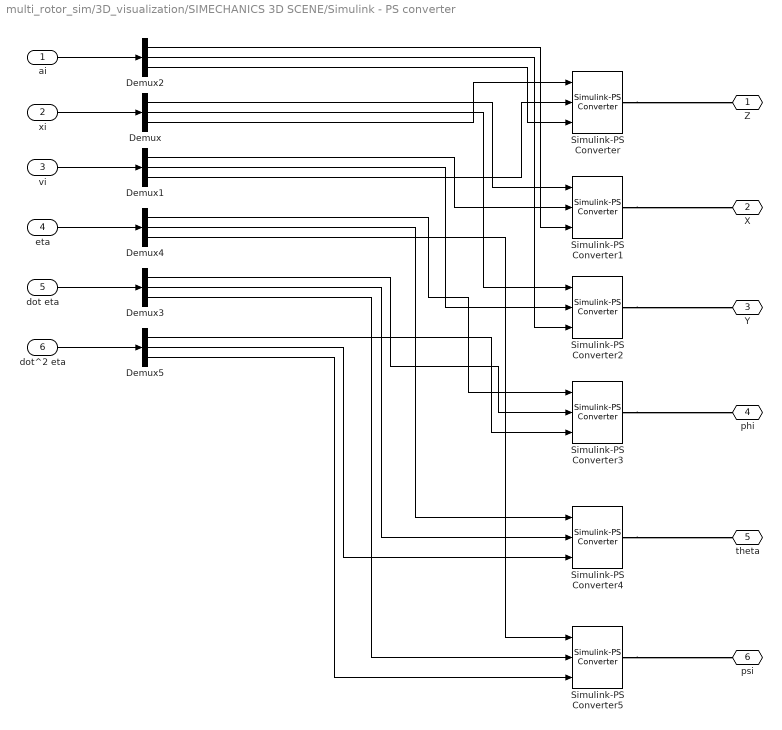
== system multi_rotor_sim/3D_visualization/SIMECHANICS 3D SCENE/Simulink - PS converter ==
  ai : Inport
  xi : Inport  Port=2
  vi : Inport  Port=3
  eta : Inport  Port=4
  dot eta : Inport  Port=5  LockScale=on
  dot^2 eta : Inport  Port=6
  Demux{,1..5} (6 alike) : Demux  Outputs=3
  Simulink-PS Converter : nesl_utility/Simulink-PS Converter  PhysicalDomain=network_engine_domain  SubClassName=ps_input  LeftPortType=input  RightPortType=output  PseudoPeriodic=off  Frequencies=[]  NoiseDistribution=none  NoiseParameters=[]  Unit=m  AffineConversion=off  FilteringAndDerivatives=provide  SimscapeFilterOrder=2  InputFilterTimeConstant=0.001  UdotUserProvided=2
  Simulink-PS Converter1 : nesl_utility/Simulink-PS Converter  PhysicalDomain=network_engine_domain  SubClassName=ps_input  LeftPortType=input  RightPortType=output  PseudoPeriodic=off  Frequencies=[]  NoiseDistribution=none  NoiseParameters=[]  Unit=m  AffineConversion=off  FilteringAndDerivatives=provide  SimscapeFilterOrder=2  InputFilterTimeConstant=0.001  UdotUserProvided=2
  Simulink-PS Converter2 : nesl_utility/Simulink-PS Converter  PhysicalDomain=network_engine_domain  SubClassName=ps_input  LeftPortType=input  RightPortType=output  PseudoPeriodic=off  Frequencies=[]  NoiseDistribution=none  NoiseParameters=[]  Unit=m  AffineConversion=off  FilteringAndDerivatives=provide  SimscapeFilterOrder=2  InputFilterTimeConstant=0.001  UdotUserProvided=2
  Simulink-PS Converter3 : nesl_utility/Simulink-PS Converter  PhysicalDomain=network_engine_domain  SubClassName=ps_input  LeftPortType=input  RightPortType=output  PseudoPeriodic=off  Frequencies=[]  NoiseDistribution=none  NoiseParameters=[]  Unit=rad  AffineConversion=off  FilteringAndDerivatives=provide  SimscapeFilterOrder=2  InputFilterTimeConstant=0.001  UdotUserProvided=2
  Simulink-PS Converter4 : nesl_utility/Simulink-PS Converter  PhysicalDomain=network_engine_domain  SubClassName=ps_input  LeftPortType=input  RightPortType=output  PseudoPeriodic=off  Frequencies=[]  NoiseDistribution=none  NoiseParameters=[]  Unit=rad  AffineConversion=off  FilteringAndDerivatives=provide  SimscapeFilterOrder=2  InputFilterTimeConstant=0.001  UdotUserProvided=2
  Simulink-PS Converter5 : nesl_utility/Simulink-PS Converter  PhysicalDomain=network_engine_domain  SubClassName=ps_input  LeftPortType=input  RightPortType=output  PseudoPeriodic=off  Frequencies=[]  NoiseDistribution=none  NoiseParameters=[]  Unit=rad  AffineConversion=off  FilteringAndDerivatives=provide  SimscapeFilterOrder=2  InputFilterTimeConstant=0.001  UdotUserProvided=2
  Z : PMIOPort  Side=Right
  X : PMIOPort  Port=2  Side=Right
  Y : PMIOPort  Port=3  Side=Right
  phi : PMIOPort  Port=4  Side=Right
  theta : PMIOPort  Port=5  Side=Right
  psi : PMIOPort  Port=6  Side=Right
  wires:
  dot^2 eta/1 -> Demux5/1
  Demux5/3 -> Simulink-PS Converter5/3
  Demux5/1 -> Simulink-PS Converter3/3
  Demux5/2 -> Simulink-PS Converter4/3
  Demux2/2 -> Simulink-PS Converter2/3
  Demux2/1 -> Simulink-PS Converter1/3
  Demux2/3 -> Simulink-PS Converter/3
  Demux1/1 -> Simulink-PS Converter1/2
  Demux1/2 -> Simulink-PS Converter2/2
  Demux/2 -> Simulink-PS Converter2/1
  Demux/1 -> Simulink-PS Converter1/1
  ai/1 -> Demux2/1
  Demux1/3 -> Simulink-PS Converter/2
  Demux/3 -> Simulink-PS Converter/1
  dot eta/1 -> Demux3/1
  xi/1 -> Demux/1
  vi/1 -> Demux1/1
  eta/1 -> Demux4/1
  Demux4/3 -> Simulink-PS Converter5/1
  Demux3/2 -> Simulink-PS Converter4/2
  Demux3/1 -> Simulink-PS Converter3/2
  Demux3/3 -> Simulink-PS Converter5/2
  Demux4/1 -> Simulink-PS Converter3/1
  Demux4/2 -> Simulink-PS Converter4/1
  connections:
  Simulink-PS Converter2/RConn1 -- Y/RConn1
  Simulink-PS Converter1/RConn1 -- X/RConn1
  Simulink-PS Converter/RConn1 -- Z/RConn1
  Simulink-PS Converter5/RConn1 -- psi/RConn1
  Simulink-PS Converter4/RConn1 -- theta/RConn1
  Simulink-PS Converter3/RConn1 -- phi/RConn1

== system multi_rotor_sim/3D_visualization/SIMECHANICS 3D SCENE/Simulink - PS converter1 ==
  xi : Inport
  vi : Inport  Port=2
  ai : Inport  Port=3
  Demux : Demux  Outputs=3
  Demux1 : Demux  Outputs=3
  Demux2 : Demux  Outputs=3
  Simulink-PS Converter : nesl_utility/Simulink-PS Converter  PhysicalDomain=network_engine_domain  SubClassName=ps_input  LeftPortType=input  RightPortType=output  PseudoPeriodic=off  Frequencies=[]  NoiseDistribution=none  NoiseParameters=[]  Unit=m  AffineConversion=off  FilteringAndDerivatives=provide  SimscapeFilterOrder=2  InputFilterTimeConstant=0.001  UdotUserProvided=2
  Simulink-PS Converter1 : nesl_utility/Simulink-PS Converter  PhysicalDomain=network_engine_domain  SubClassName=ps_input  LeftPortType=input  RightPortType=output  PseudoPeriodic=off  Frequencies=[]  NoiseDistribution=none  NoiseParameters=[]  Unit=m  AffineConversion=off  FilteringAndDerivatives=provide  SimscapeFilterOrder=2  InputFilterTimeConstant=0.001  UdotUserProvided=2
  Simulink-PS Converter2 : nesl_utility/Simulink-PS Converter  PhysicalDomain=network_engine_domain  SubClassName=ps_input  LeftPortType=input  RightPortType=output  PseudoPeriodic=off  Frequencies=[]  NoiseDistribution=none  NoiseParameters=[]  Unit=m  AffineConversion=off  FilteringAndDerivatives=provide  SimscapeFilterOrder=2  InputFilterTimeConstant=0.001  UdotUserProvided=2
  Z : PMIOPort  Side=Right
  X : PMIOPort  Port=2  Side=Right
  Y : PMIOPort  Port=3  Side=Right
  wires:
  vi/1 -> Demux1/1
  xi/1 -> Demux/1
  Demux/3 -> Simulink-PS Converter/1
  Demux1/3 -> Simulink-PS Converter/2
  ai/1 -> Demux2/1
  Demux/1 -> Simulink-PS Converter1/1
  Demux/2 -> Simulink-PS Converter2/1
  Demux1/2 -> Simulink-PS Converter2/2
  Demux1/1 -> Simulink-PS Converter1/2
  Demux2/3 -> Simulink-PS Converter/3
  Demux2/1 -> Simulink-PS Converter1/3
  Demux2/2 -> Simulink-PS Converter2/3
  connections:
  Simulink-PS Converter/RConn1 -- Z/RConn1
  Simulink-PS Converter1/RConn1 -- X/RConn1
  Simulink-PS Converter2/RConn1 -- Y/RConn1

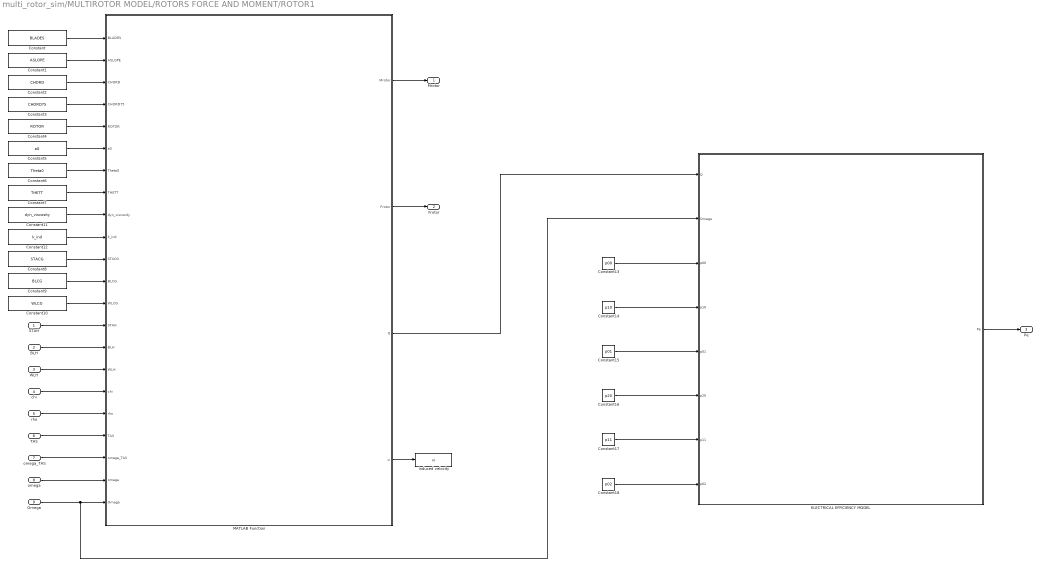
== system multi_rotor_sim/MULTIROTOR MODEL/ROTORS FORCE AND MOMENT/ROTOR1 ==
  STAH : Inport
  BLH : Inport  Port=2
  WLH : Inport  Port=3
  chi : Inport  Port=4
  rho : Inport  Port=5
  TAS : Inport  Port=6
  omega_TAS : Inport  Port=7
  omega : Inport  Port=8
  Omega : Inport  Port=9
  Constant : Constant  Value=BLADES
  Constant1 : Constant  Value=ASLOPE
  Constant10 : Constant  Value=WLCG
  Constant11 : Constant  Value=dyn_viscosity
  Constant12 : Constant  Value=k_ind
  Constant13 : Constant  Value=p00
  Constant14 : Constant  Value=p10
  Constant15 : Constant  Value=p01
  Constant16 : Constant  Value=p20
  Constant17 : Constant  Value=p11
  Constant18 : Constant  Value=p02
  Constant2 : Constant  Value=CHORD
  Constant3 : Constant  Value=CHORD75
  Constant4 : Constant  Value=ROTOR
  Constant5 : Constant  Value=a0
  Constant6 : Constant  Value=Theta0
  Constant7 : Constant  Value=THETT
  Constant8 : Constant  Value=STACG
  Constant9 : Constant  Value=BLCG
  ELECTRICAL EFFICIENCY MODEL : MATLAB Function  TreatAsAtomicUnit=on
  MATLAB Function : MATLAB Function  TreatAsAtomicUnit=on
  induced velocity : ToWorkspace  VariableName=vi  SampleTime=-1
  Mrotor : Outport
  Frotor : Outport  Port=2
  Pe : Outport  Port=3
  wires:
  MATLAB Function/3(Q) -> ELECTRICAL EFFICIENCY MODEL/1(Q)
  omega_TAS/1 -> MATLAB Function/20(omega_TAS)
  Constant16/1 -> ELECTRICAL EFFICIENCY MODEL/6(p20)
  Omega/1 -> ELECTRICAL EFFICIENCY MODEL/2(Omega), MATLAB Function/22(Omega)
  Constant13/1 -> ELECTRICAL EFFICIENCY MODEL/3(p00)
  Constant14/1 -> ELECTRICAL EFFICIENCY MODEL/4(p10)
  BLH/1 -> MATLAB Function/15(BLH)
  Constant3/1 -> MATLAB Function/4(CHORD75)
  Constant/1 -> MATLAB Function/1(BLADES)
  Constant17/1 -> ELECTRICAL EFFICIENCY MODEL/7(p11)
  Constant18/1 -> ELECTRICAL EFFICIENCY MODEL/8(p02)
  Constant15/1 -> ELECTRICAL EFFICIENCY MODEL/5(p01)
  Constant8/1 -> MATLAB Function/11(STACG)
  STAH/1 -> MATLAB Function/14(STAH)
  Constant6/1 -> MATLAB Function/7(Theta0)
  Constant1/1 -> MATLAB Function/2(ASLOPE)
  Constant4/1 -> MATLAB Function/5(ROTOR)
  Constant5/1 -> MATLAB Function/6(a0)
  Constant12/1 -> MATLAB Function/10(k_ind)
  WLH/1 -> MATLAB Function/16(WLH)
  chi/1 -> MATLAB Function/17(chi)
  TAS/1 -> MATLAB Function/19(TAS)
  Constant7/1 -> MATLAB Function/8(THETT)
  omega/1 -> MATLAB Function/21(omega)
  Constant2/1 -> MATLAB Function/3(CHORD)
  Constant11/1 -> MATLAB Function/9(dyn_viscosity)
  rho/1 -> MATLAB Function/18(rho)
  MATLAB Function/1(Mrotor) -> Mrotor/1
  Constant10/1 -> MATLAB Function/13(WLCG)
  Constant9/1 -> MATLAB Function/12(BLCG)
  MATLAB Function/2(Frotor) -> Frotor/1
  ELECTRICAL EFFICIENCY MODEL/1(Pe) -> Pe/1
  MATLAB Function/4(vi) -> induced velocity/1

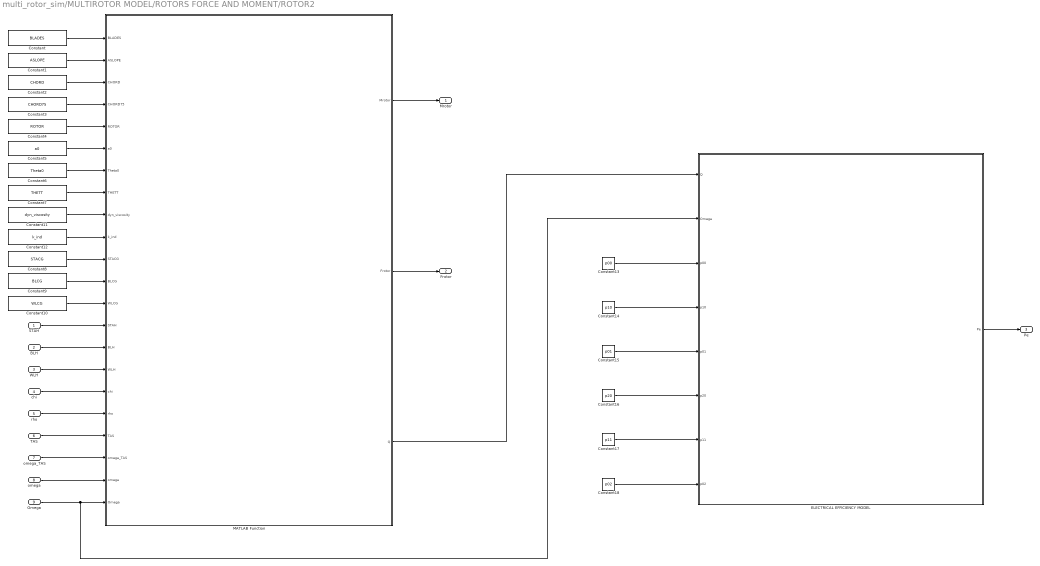
== system multi_rotor_sim/MULTIROTOR MODEL/ROTORS FORCE AND MOMENT/ROTOR2 ==
  STAH : Inport
  BLH : Inport  Port=2
  WLH : Inport  Port=3
  chi : Inport  Port=4
  rho : Inport  Port=5
  TAS : Inport  Port=6
  omega_TAS : Inport  Port=7
  omega : Inport  Port=8
  Omega : Inport  Port=9
  Constant : Constant  Value=BLADES
  Constant1 : Constant  Value=ASLOPE
  Constant10 : Constant  Value=WLCG
  Constant11 : Constant  Value=dyn_viscosity
  Constant12 : Constant  Value=k_ind
  Constant13 : Constant  Value=p00
  Constant14 : Constant  Value=p10
  Constant15 : Constant  Value=p01
  Constant16 : Constant  Value=p20
  Constant17 : Constant  Value=p11
  Constant18 : Constant  Value=p02
  Constant2 : Constant  Value=CHORD
  Constant3 : Constant  Value=CHORD75
  Constant4 : Constant  Value=ROTOR
  Constant5 : Constant  Value=a0
  Constant6 : Constant  Value=Theta0
  Constant7 : Constant  Value=THETT
  Constant8 : Constant  Value=STACG
  Constant9 : Constant  Value=BLCG
  ELECTRICAL EFFICIENCY MODEL : MATLAB Function  TreatAsAtomicUnit=on
  MATLAB Function : MATLAB Function  TreatAsAtomicUnit=on
  Mrotor : Outport
  Frotor : Outport  Port=2
  Pe : Outport  Port=3
  wires:
  MATLAB Function/3(Q) -> ELECTRICAL EFFICIENCY MODEL/1(Q)
  omega_TAS/1 -> MATLAB Function/20(omega_TAS)
  Constant16/1 -> ELECTRICAL EFFICIENCY MODEL/6(p20)
  Omega/1 -> ELECTRICAL EFFICIENCY MODEL/2(Omega), MATLAB Function/22(Omega)
  Constant13/1 -> ELECTRICAL EFFICIENCY MODEL/3(p00)
  Constant14/1 -> ELECTRICAL EFFICIENCY MODEL/4(p10)
  BLH/1 -> MATLAB Function/15(BLH)
  Constant3/1 -> MATLAB Function/4(CHORD75)
  Constant/1 -> MATLAB Function/1(BLADES)
  Constant17/1 -> ELECTRICAL EFFICIENCY MODEL/7(p11)
  Constant18/1 -> ELECTRICAL EFFICIENCY MODEL/8(p02)
  Constant15/1 -> ELECTRICAL EFFICIENCY MODEL/5(p01)
  Constant8/1 -> MATLAB Function/11(STACG)
  STAH/1 -> MATLAB Function/14(STAH)
  Constant6/1 -> MATLAB Function/7(Theta0)
  Constant1/1 -> MATLAB Function/2(ASLOPE)
  Constant4/1 -> MATLAB Function/5(ROTOR)
  Constant5/1 -> MATLAB Function/6(a0)
  Constant12/1 -> MATLAB Function/10(k_ind)
  WLH/1 -> MATLAB Function/16(WLH)
  chi/1 -> MATLAB Function/17(chi)
  TAS/1 -> MATLAB Function/19(TAS)
  Constant7/1 -> MATLAB Function/8(THETT)
  omega/1 -> MATLAB Function/21(omega)
  Constant2/1 -> MATLAB Function/3(CHORD)
  Constant11/1 -> MATLAB Function/9(dyn_viscosity)
  rho/1 -> MATLAB Function/18(rho)
  MATLAB Function/1(Mrotor) -> Mrotor/1
  Constant10/1 -> MATLAB Function/13(WLCG)
  Constant9/1 -> MATLAB Function/12(BLCG)
  MATLAB Function/2(Frotor) -> Frotor/1
  ELECTRICAL EFFICIENCY MODEL/1(Pe) -> Pe/1

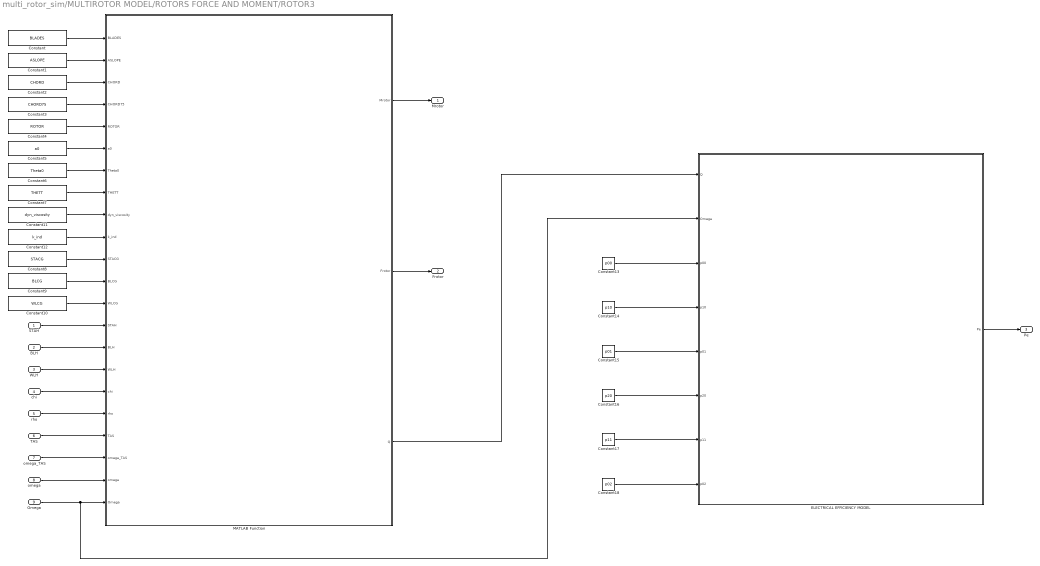
== system multi_rotor_sim/MULTIROTOR MODEL/ROTORS FORCE AND MOMENT/ROTOR3 ==
  STAH : Inport
  BLH : Inport  Port=2
  WLH : Inport  Port=3
  chi : Inport  Port=4
  rho : Inport  Port=5
  TAS : Inport  Port=6
  omega_TAS : Inport  Port=7
  omega : Inport  Port=8
  Omega : Inport  Port=9
  Constant : Constant  Value=BLADES
  Constant1 : Constant  Value=ASLOPE
  Constant10 : Constant  Value=WLCG
  Constant11 : Constant  Value=dyn_viscosity
  Constant12 : Constant  Value=k_ind
  Constant13 : Constant  Value=p00
  Constant14 : Constant  Value=p10
  Constant15 : Constant  Value=p01
  Constant16 : Constant  Value=p20
  Constant17 : Constant  Value=p11
  Constant18 : Constant  Value=p02
  Constant2 : Constant  Value=CHORD
  Constant3 : Constant  Value=CHORD75
  Constant4 : Constant  Value=ROTOR
  Constant5 : Constant  Value=a0
  Constant6 : Constant  Value=Theta0
  Constant7 : Constant  Value=THETT
  Constant8 : Constant  Value=STACG
  Constant9 : Constant  Value=BLCG
  ELECTRICAL EFFICIENCY MODEL : MATLAB Function  TreatAsAtomicUnit=on
  MATLAB Function : MATLAB Function  TreatAsAtomicUnit=on
  Mrotor : Outport
  Frotor : Outport  Port=2
  Pe : Outport  Port=3
  wires:
  MATLAB Function/3(Q) -> ELECTRICAL EFFICIENCY MODEL/1(Q)
  omega_TAS/1 -> MATLAB Function/20(omega_TAS)
  Constant16/1 -> ELECTRICAL EFFICIENCY MODEL/6(p20)
  Omega/1 -> ELECTRICAL EFFICIENCY MODEL/2(Omega), MATLAB Function/22(Omega)
  Constant13/1 -> ELECTRICAL EFFICIENCY MODEL/3(p00)
  Constant14/1 -> ELECTRICAL EFFICIENCY MODEL/4(p10)
  BLH/1 -> MATLAB Function/15(BLH)
  Constant3/1 -> MATLAB Function/4(CHORD75)
  Constant/1 -> MATLAB Function/1(BLADES)
  Constant17/1 -> ELECTRICAL EFFICIENCY MODEL/7(p11)
  Constant18/1 -> ELECTRICAL EFFICIENCY MODEL/8(p02)
  Constant15/1 -> ELECTRICAL EFFICIENCY MODEL/5(p01)
  Constant8/1 -> MATLAB Function/11(STACG)
  STAH/1 -> MATLAB Function/14(STAH)
  Constant6/1 -> MATLAB Function/7(Theta0)
  Constant1/1 -> MATLAB Function/2(ASLOPE)
  Constant4/1 -> MATLAB Function/5(ROTOR)
  Constant5/1 -> MATLAB Function/6(a0)
  Constant12/1 -> MATLAB Function/10(k_ind)
  WLH/1 -> MATLAB Function/16(WLH)
  chi/1 -> MATLAB Function/17(chi)
  TAS/1 -> MATLAB Function/19(TAS)
  Constant7/1 -> MATLAB Function/8(THETT)
  omega/1 -> MATLAB Function/21(omega)
  Constant2/1 -> MATLAB Function/3(CHORD)
  Constant11/1 -> MATLAB Function/9(dyn_viscosity)
  rho/1 -> MATLAB Function/18(rho)
  MATLAB Function/1(Mrotor) -> Mrotor/1
  Constant10/1 -> MATLAB Function/13(WLCG)
  Constant9/1 -> MATLAB Function/12(BLCG)
  MATLAB Function/2(Frotor) -> Frotor/1
  ELECTRICAL EFFICIENCY MODEL/1(Pe) -> Pe/1

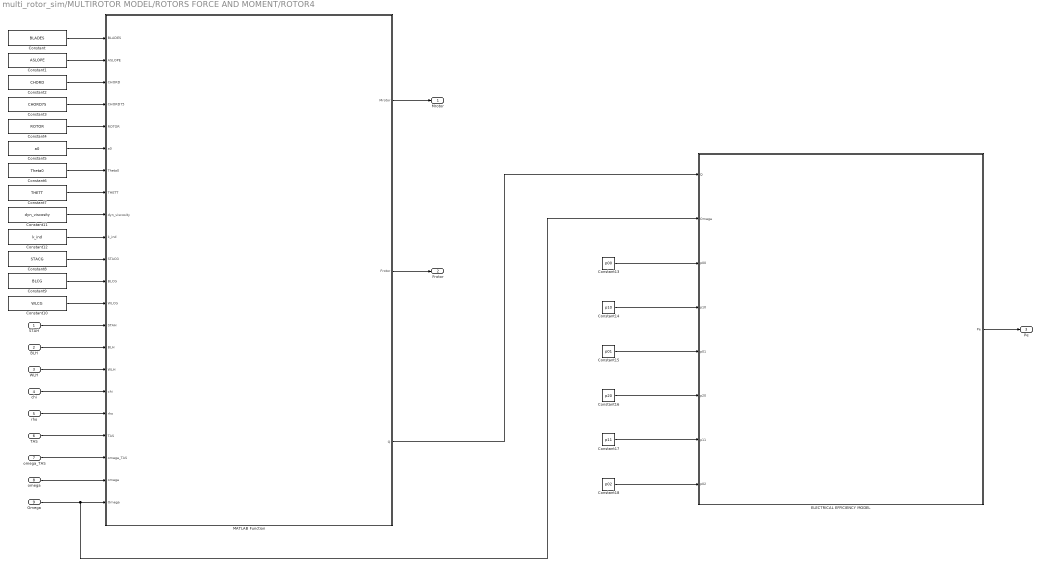
== system multi_rotor_sim/MULTIROTOR MODEL/ROTORS FORCE AND MOMENT/ROTOR4 ==
  STAH : Inport
  BLH : Inport  Port=2
  WLH : Inport  Port=3
  chi : Inport  Port=4
  rho : Inport  Port=5
  TAS : Inport  Port=6
  omega_TAS : Inport  Port=7
  omega : Inport  Port=8
  Omega : Inport  Port=9
  Constant : Constant  Value=BLADES
  Constant1 : Constant  Value=ASLOPE
  Constant10 : Constant  Value=WLCG
  Constant11 : Constant  Value=dyn_viscosity
  Constant12 : Constant  Value=k_ind
  Constant13 : Constant  Value=p00
  Constant14 : Constant  Value=p10
  Constant15 : Constant  Value=p01
  Constant16 : Constant  Value=p20
  Constant17 : Constant  Value=p11
  Constant18 : Constant  Value=p02
  Constant2 : Constant  Value=CHORD
  Constant3 : Constant  Value=CHORD75
  Constant4 : Constant  Value=ROTOR
  Constant5 : Constant  Value=a0
  Constant6 : Constant  Value=Theta0
  Constant7 : Constant  Value=THETT
  Constant8 : Constant  Value=STACG
  Constant9 : Constant  Value=BLCG
  ELECTRICAL EFFICIENCY MODEL : MATLAB Function  TreatAsAtomicUnit=on
  MATLAB Function : MATLAB Function  TreatAsAtomicUnit=on
  Mrotor : Outport
  Frotor : Outport  Port=2
  Pe : Outport  Port=3
  wires:
  MATLAB Function/3(Q) -> ELECTRICAL EFFICIENCY MODEL/1(Q)
  omega_TAS/1 -> MATLAB Function/20(omega_TAS)
  Constant16/1 -> ELECTRICAL EFFICIENCY MODEL/6(p20)
  Omega/1 -> ELECTRICAL EFFICIENCY MODEL/2(Omega), MATLAB Function/22(Omega)
  Constant13/1 -> ELECTRICAL EFFICIENCY MODEL/3(p00)
  Constant14/1 -> ELECTRICAL EFFICIENCY MODEL/4(p10)
  BLH/1 -> MATLAB Function/15(BLH)
  Constant3/1 -> MATLAB Function/4(CHORD75)
  Constant/1 -> MATLAB Function/1(BLADES)
  Constant17/1 -> ELECTRICAL EFFICIENCY MODEL/7(p11)
  Constant18/1 -> ELECTRICAL EFFICIENCY MODEL/8(p02)
  Constant15/1 -> ELECTRICAL EFFICIENCY MODEL/5(p01)
  Constant8/1 -> MATLAB Function/11(STACG)
  STAH/1 -> MATLAB Function/14(STAH)
  Constant6/1 -> MATLAB Function/7(Theta0)
  Constant1/1 -> MATLAB Function/2(ASLOPE)
  Constant4/1 -> MATLAB Function/5(ROTOR)
  Constant5/1 -> MATLAB Function/6(a0)
  Constant12/1 -> MATLAB Function/10(k_ind)
  WLH/1 -> MATLAB Function/16(WLH)
  chi/1 -> MATLAB Function/17(chi)
  TAS/1 -> MATLAB Function/19(TAS)
  Constant7/1 -> MATLAB Function/8(THETT)
  omega/1 -> MATLAB Function/21(omega)
  Constant2/1 -> MATLAB Function/3(CHORD)
  Constant11/1 -> MATLAB Function/9(dyn_viscosity)
  rho/1 -> MATLAB Function/18(rho)
  MATLAB Function/1(Mrotor) -> Mrotor/1
  Constant10/1 -> MATLAB Function/13(WLCG)
  Constant9/1 -> MATLAB Function/12(BLCG)
  MATLAB Function/2(Frotor) -> Frotor/1
  ELECTRICAL EFFICIENCY MODEL/1(Pe) -> Pe/1
